simulink model "StaticStabilityMarginLong_TestModel"  (R2014a)
settings: Solver=ode45  StartTime=0.0  StopTime=10.0  RelTol=1e-3
libraries: rocket_angular_flight_library x1
settings Model: Creator=scorpii  LastModifiedBy=scorpii

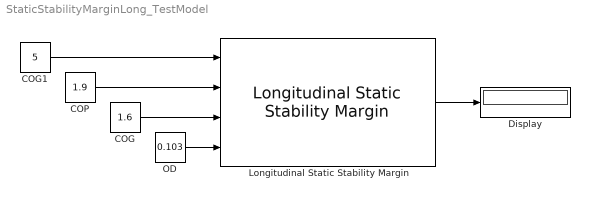
== system StaticStabilityMarginLong_TestModel ==
  COG : Constant  Value=1.6
  COG1 : Constant  Value=5
  COP : Constant  Value=1.9
  Display : Display
  Longitudinal Static Stability Margin : rocket_angular_flight_library/Longitudinal Static Stability Margin
  OD : Constant  Value=0.103
  wires:
  COP/1 -> Longitudinal Static Stability Margin/2
  COG/1 -> Longitudinal Static Stability Margin/3
  OD/1 -> Longitudinal Static Stability Margin/4
  COG1/1 -> Longitudinal Static Stability Margin/1
  Longitudinal Static Stability Margin/1 -> Display/1
